simulink model "multidrivesystem"  (R2020a)
settings: Solver=ode23  StartTime=0.0  StopTime=1  MaxStep=20  RelTol=1e-4
libraries: powerlib x250
(part 1 of 2)
settings Model: Creator=shalakasitre  LastModifiedBy=shalakasitre
settings DataIOCC: ReturnWorkspaceOutputs=off

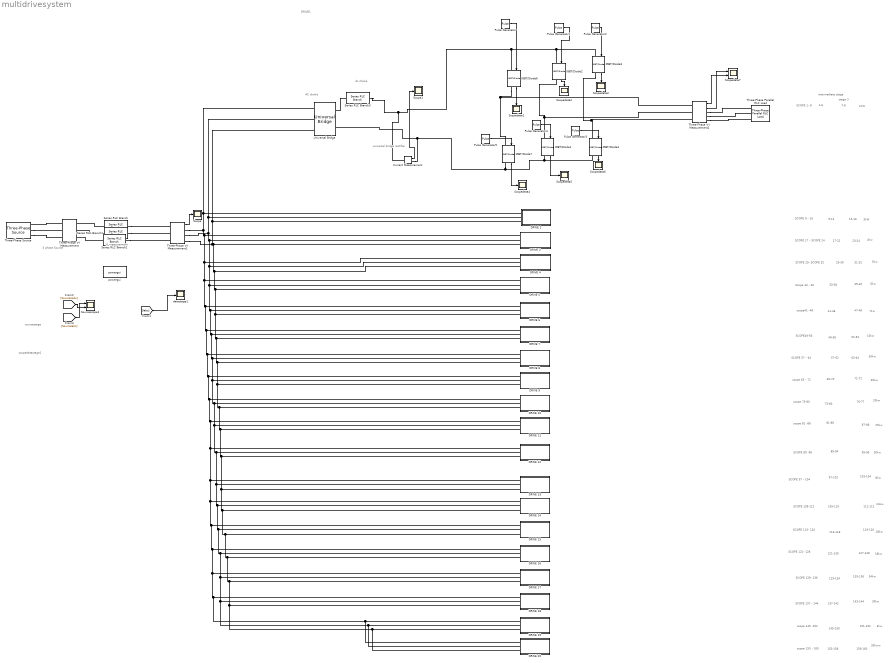
== system multidrivesystem ==
  note: DRIVE1
  note: 30kww
  note: 3kw
  note: 30kw
  note: 34kw
  note: 18kw
  note: 28kw
  note: 24kw
  note: 8kw
  note: 30kw
  note: 25kw
  note: 20kw
  note: 30kw
  note: 30kw
  note: 10kw
  note: 7kw
  note: 6kw
  note: 5kw
  note: 4kw
  note: 3kW
  note: 1kW
  note: 1-6
  note: 153-158
  note: 145-150
  note: 137-142
  note: 129-134
  note: 121-126
  note: 113-118
  note: 105-110
  note: 97-102
  note: 89-94
  note: 81-86
  note: 73-80
  note: 65-70
  note: 57-62
  note: 49-56
  note: 41-46
  note: 33-38
  note: 25-30
  note: 17-22
  note: 9-14
  note: 159-160
  note: 151-152
  note: 143-144
  note: 135-136
  note: 127-128
  note: 119-120
  note: 111-112
  note: 103-104
  note: 95-96
  note: 87-88
  note: 76-77
  note: 71-72
  note: 63-64
  note: 52-53
  note: 47-48
  note: 39-40
  note: 31-32
  note: 23-24
  note: 15-16
  note: intermediate
      | stage
  note: stage 3
  note: sourcestage
  note: scopedatastage1
  note: 7-8
  note: scope 153 - 160
  note: scope 145 -152
  note: SCOPE 137 - 144
  note: SCOPE 129- 136
  note: SCOPE 121- 128
  note: SCOPE 113- 120
  note: SCOPE 105-112
  note: SCOPE 97 - 104
  note: SCOPE 89 -96
  note: scope 81 -88
  note: scope 73-80
  note: scope 65 - 72
  note: SCOPE 57 - 64
  note: scope41- 48
  note: Scope 33 - 40
  note: SCOPE49-56
  note: SCOPE 1- 8
  note: SCOPE 9 - 16
  note: SCOPE 17 - SCOPE 24
  note: SCOPE 25- SCOPE 32
  note: 3 phase Source
  note: VI measurement
  note: universal bridge rectifier
  note: AC choke
  note: dc choke
  Current Measurement : powerlib/Measurements/Current Measurement  PhasorSimulation=off  OutputType=Complex  PSBequivalent=0
  DRIVE 10 : Subsystem
  DRIVE 11 : Subsystem
  DRIVE 12 : Subsystem
  DRIVE 13 : Subsystem
  DRIVE 14 : Subsystem
  DRIVE 15 : Subsystem
  DRIVE 16 : Subsystem
  DRIVE 17 : Subsystem
  DRIVE 18 : Subsystem
  DRIVE 19 : Subsystem
  DRIVE 2 : Subsystem
  DRIVE 20 : Subsystem
  DRIVE 3 : Subsystem
      mask init:
      | set_param(gcb,'LinkStatus','none');
  DRIVE 4 : Subsystem
      mask init:
      | set_param(gcb,'LinkStatus','none');
  DRIVE 5 : Subsystem
  DRIVE 6 : Subsystem
  "DRIVE 7 " : Subsystem
  DRIVE 8 : Subsystem
  DRIVE 9 : Subsystem
  IGBT/Diode{1..4,6..7} (6 alike) : powerlib/Power Electronics/IGBT//Diode  Ron=1e-3  Rs=1e5  Cs=inf  Measurements=on
  Pulse Generator{,1..5} (6 alike) : DiscretePulseGenerator  PulseType=Time based  Period=10  PulseWidth=5
  Scope : Scope
  Scope1 : Scope
  Scopedata{1..6} (6 alike) : Scope
  Scopedata7 : Scope  NumInputPorts=2
  Series RLC Branch : powerlib/Elements/Series RLC Branch  LConnTagsString=__new0  RConnTagsString=__new0  BranchType=L  Resistance=1  Inductance=150e-6  SetiL0=off  InitialCurrent=0  Capacitance=1e-6  Setx0=off  InitialVoltage=0  Measurements=None
  Series RLC Branch1 : powerlib/Elements/Series RLC Branch  LConnTagsString=__new0  RConnTagsString=__new0  BranchType=L  Resistance=1  Inductance=150e-6  SetiL0=off  InitialCurrent=0  Capacitance=1e-6  Setx0=off  InitialVoltage=0  Measurements=None
  Series RLC Branch2 : powerlib/Elements/Series RLC Branch  LConnTagsString=__new0  RConnTagsString=__new0  BranchType=L  Resistance=1  Inductance=150e-6  SetiL0=off  InitialCurrent=0  Capacitance=1e-6  Setx0=off  InitialVoltage=0  Measurements=None
  Series RLC Branch3 : powerlib/Elements/Series RLC Branch  LConnTagsString=__new0  RConnTagsString=__new0  BranchType=L  Resistance=1  Inductance=3e-3  SetiL0=off  InitialCurrent=0  Capacitance=1e-6  Setx0=off  InitialVoltage=0  Measurements=None
  Sourcescope1 : Scope  NumInputPorts=2
  Three-Phase Parallel RLC Load : powerlib/Elements/Three-Phase Parallel RLC Load  LConnTagsString=A|B|C  Configuration=Y (grounded)  NominalVoltage=1000  Vabc=[1e3 1e3 1e3]  Vabcp=[1e3 1e3 1e3]  NominalFrequency=60  UnbalancedPower=off  ActivePower=5e3  InductivePower=0  CapacitivePower=0  Pabc=[10e3 9e3 11e3]  QLabc=[100 90 110]  QCabc=[100 90 110]  Pabcp=[10e3 9e3 11e3]  QLabcp=[100 90 110]  QCabcp=[100 90 110]  Measurements=None  LoadType=constant Z
  Three-Phase V-I Measurement : powerlib/Measurements/Three-Phase V-I Measurement  VoltageMeasurement=phase-to-ground  SetLabelV=on  LabelV=SourceVabc  Vpu=off  VpuLL=off  CurrentMeasurement=yes  SetLabelI=on  LabelI=SourceIabc  Ipu=off  Pbase=100e6  Vbase=500e3  OutputType=Complex  PhasorSimulation=off  PSBequivalent=0
  Three-Phase V-I Measurement1 : powerlib/Measurements/Three-Phase V-I Measurement  VoltageMeasurement=phase-to-ground  SetLabelV=off  LabelV=Vabc  Vpu=off  VpuLL=off  CurrentMeasurement=yes  SetLabelI=on  LabelI=Iabc  Ipu=off  Pbase=100e6  Vbase=500e3  OutputType=Complex  PhasorSimulation=off  PSBequivalent=0
  Three-Phase V-I Measurement2 : powerlib/Measurements/Three-Phase V-I Measurement  VoltageMeasurement=phase-to-ground  SetLabelV=off  LabelV=Vabc  Vpu=off  VpuLL=off  CurrentMeasurement=yes  SetLabelI=off  LabelI=Iabc  Ipu=off  Pbase=100e6  Vbase=500e3  OutputType=Complex  PhasorSimulation=off  PSBequivalent=0
  Three-Phase Source : powerlib/Electrical Sources/Three-Phase Source  InternalConnection=Yg  VoltagePhases=off  Voltage=440  PhaseAngle=0  Voltage_phases=[25e3 25e3 25e3]/sqrt(3)  PhaseAngles_phases=[0 -120 +120]  Frequency=60  NonIdealSource=off  SpecifyImpedance=off  Resistance=0  Inductance=0  ShortCircuitLevel=100e6  BaseVoltage=25e3  XRratio=7  BusType=swing  Pref=10e3  Qref=0  Prefabc=[10e3, 10e3, 10e3]  Qrefabc=[0, 0, 0]  Qmin=-inf  Qmax=inf
  Universal Bridge : powerlib/Power Electronics/Universal Bridge  Arms=3  SnubberResistance=1e5  SnubberCapacitance=inf  Device=Diodes  Ron=1e-3  Lon=0  ForwardVoltages="[  0  0  ]"  ForwardVoltage=0  GTOparameters=[ 10e-6 , 20e-6 ]  IGBTparameters=[ 1e-6 , 2e-6 ]  Measurements=None  Measurements_2=None  converterType=Rectifier
  datastage1 : Scope
  powergui : powerlib/powergui  Priority=1  SimulationMode=Discrete  SampleTime=50e-6  frequency=60  Iterations=50  frequencyindice=0  Pbase=100e6  ErrMax=1e-4  UnitsV=kV  UnitsW=MW  buscounter=0  FunctionMessages=off  echomessages=off  EnableUseOfTLC=off  CurrentSourceSwitches=off  DisableSnubberDevices=off  DisableRonSwitches=off  DisableVfSwitches=off  DisplayEquations=off  AutomaticDiscreteSolvers=off  SolverType=Tustin/Backward Euler (TBE)  Interpol=off  ExternalGateDelay=off  methode=off  Ts=100  x0status=blocks  SPID=on  SwTol=0  HookPort=off  NonlinearTolerance=1e-4  nMaxIteration=100  ContinueOnMaxIteration=off  RestoreLinks=warning  ResistiveCurrentMeasurement=off  Frange=[0:2:500]  Ylog=off  Xlog=on  ShowGrid=off  save=off  variable=ZData  structure=Drive1_stage2voltage  ZoomFFT=off  StartTime=0  cycles=1  DisplayStyle=2  fundamental=60  FreqAxis=off  MaxFrequency=1000  frequencyindicesteady=1  RmsSteady=1  display=off
  wires:
  [Iabc] -> datastage1/1
  [SourceVabc] -> Sourcescope1/2
  [SourceIabc] -> Sourcescope1/1
  Three-Phase V-I Measurement1/1 -> Scope/1
  Three-Phase V-I Measurement2/1 -> Scopedata7/2
  Current Measurement/1 -> Scope1/1
  IGBT/Diode1/1 -> Scopedata5/1
  IGBT/Diode3/1 -> Scopedata3/1
  Pulse Generator1/1 -> IGBT/Diode2/1
  Three-Phase V-I Measurement2/2 -> Scopedata7/1
  Pulse Generator2/1 -> IGBT/Diode3/1
  IGBT/Diode4/1 -> Scopedata6/1
  Pulse Generator5/1 -> IGBT/Diode7/1
  Pulse Generator4/1 -> IGBT/Diode1/1
  IGBT/Diode7/1 -> Scopedata4/1
  IGBT/Diode6/1 -> Scopedata1/1
  IGBT/Diode2/1 -> Scopedata2/1
  Pulse Generator/1 -> IGBT/Diode6/1
  Pulse Generator3/1 -> IGBT/Diode4/1
  connections:
  Three-Phase V-I Measurement/LConn1 -- Three-Phase Source/RConn1
  Three-Phase Source/RConn2 -- Three-Phase V-I Measurement/LConn2
  Three-Phase Source/RConn3 -- Three-Phase V-I Measurement/LConn3
  Series RLC Branch/LConn1 -- Three-Phase V-I Measurement/RConn1
  Series RLC Branch1/LConn1 -- Three-Phase V-I Measurement/RConn2
  Series RLC Branch2/LConn1 -- Three-Phase V-I Measurement/RConn3
  DRIVE 20/LConn3 -- DRIVE 19/LConn3 -- DRIVE 18/LConn3 -- DRIVE 17/LConn3 -- DRIVE 16/LConn3 -- DRIVE 15/LConn3 -- DRIVE 14/LConn3 -- DRIVE 13/LConn3 -- DRIVE 12/LConn3 -- DRIVE 11/LConn3 -- DRIVE 10/LConn3 -- DRIVE 9/LConn3 -- DRIVE 8/LConn3 -- "DRIVE 7 "/LConn3 -- DRIVE 6/LConn3 -- DRIVE 5/LConn3 -- DRIVE 4/LConn3 -- DRIVE 3/LConn3 -- Three-Phase V-I Measurement1/RConn3 -- Universal Bridge/LConn3 -- DRIVE 2/LConn3
  DRIVE 20/LConn1 -- DRIVE 19/LConn1 -- DRIVE 18/LConn1 -- DRIVE 17/LConn1 -- DRIVE 16/LConn1 -- DRIVE 15/LConn1 -- DRIVE 14/LConn1 -- DRIVE 13/LConn1 -- DRIVE 12/LConn1 -- DRIVE 11/LConn1 -- DRIVE 10/LConn1 -- DRIVE 9/LConn1 -- DRIVE 8/LConn1 -- "DRIVE 7 "/LConn1 -- DRIVE 6/LConn1 -- DRIVE 5/LConn1 -- Universal Bridge/LConn1 -- DRIVE 2/LConn1 -- Three-Phase V-I Measurement1/RConn1 -- DRIVE 3/LConn1 -- DRIVE 4/LConn1
  Universal Bridge/LConn2 -- DRIVE 2/LConn2 -- DRIVE 20/LConn2 -- DRIVE 19/LConn2 -- DRIVE 18/LConn2 -- DRIVE 17/LConn2 -- DRIVE 16/LConn2 -- DRIVE 15/LConn2 -- DRIVE 14/LConn2 -- DRIVE 13/LConn2 -- DRIVE 12/LConn2 -- DRIVE 11/LConn2 -- DRIVE 10/LConn2 -- DRIVE 9/LConn2 -- DRIVE 8/LConn2 -- "DRIVE 7 "/LConn2 -- DRIVE 6/LConn2 -- DRIVE 5/LConn2 -- DRIVE 4/LConn2 -- DRIVE 3/LConn2 -- Three-Phase V-I Measurement1/RConn2
  Series RLC Branch/RConn1 -- Three-Phase V-I Measurement1/LConn1
  Series RLC Branch1/RConn1 -- Three-Phase V-I Measurement1/LConn2
  Series RLC Branch2/RConn1 -- Three-Phase V-I Measurement1/LConn3
  Series RLC Branch3/LConn1 -- Universal Bridge/RConn1
  IGBT/Diode3/LConn1 -- Series RLC Branch3/RConn1 -- Current Measurement/LConn1 -- IGBT/Diode6/LConn1 -- IGBT/Diode2/LConn1
  Current Measurement/RConn1 -- IGBT/Diode4/RConn1 -- IGBT/Diode1/RConn1 -- IGBT/Diode7/RConn1 -- Universal Bridge/RConn2
  IGBT/Diode3/RConn1 -- Three-Phase V-I Measurement2/LConn3 -- IGBT/Diode4/LConn1
  Three-Phase V-I Measurement2/RConn1 -- Three-Phase Parallel RLC Load/LConn1
  IGBT/Diode2/RConn1 -- Three-Phase V-I Measurement2/LConn2 -- IGBT/Diode1/LConn1
  IGBT/Diode6/RConn1 -- Three-Phase V-I Measurement2/LConn1 -- IGBT/Diode7/LConn1
  Three-Phase V-I Measurement2/RConn3 -- Three-Phase Parallel RLC Load/LConn3
  Three-Phase V-I Measurement2/RConn2 -- Three-Phase Parallel RLC Load/LConn2

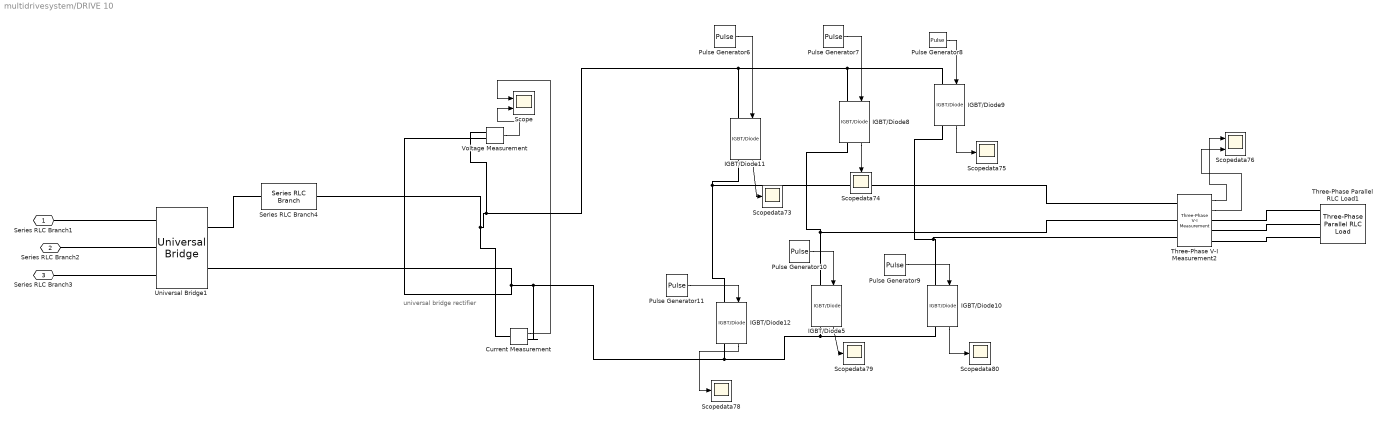
== system multidrivesystem/DRIVE 10 ==
  note: universal bridge rectifier
  Current Measurement : powerlib/Measurements/Current Measurement  PhasorSimulation=off  OutputType=Complex  PSBequivalent=0
  IGBT/Diode{5,8..12} (6 alike) : powerlib/Power Electronics/IGBT//Diode  Ron=1e-3  Rs=1e5  Cs=inf  Measurements=on
  Pulse Generator{6..11} (6 alike) : DiscretePulseGenerator  PulseType=Time based  Period=10  PulseWidth=5
  Scope : Scope  NumInputPorts=2
  Scopedata{73..75,78..80} (6 alike) : Scope
  Scopedata76 : Scope  NumInputPorts=2
  Series RLC Branch4 : powerlib/Elements/Series RLC Branch  LConnTagsString=__new0  RConnTagsString=__new0  BranchType=L  Resistance=1  Inductance=3e-3  SetiL0=off  InitialCurrent=0  Capacitance=1e-6  Setx0=off  InitialVoltage=0  Measurements=None
  Three-Phase Parallel RLC Load1 : powerlib/Elements/Three-Phase Parallel RLC Load  LConnTagsString=A|B|C  Configuration=Y (grounded)  NominalVoltage=1000  Vabc=[1e3 1e3 1e3]  Vabcp=[1e3 1e3 1e3]  NominalFrequency=60  UnbalancedPower=off  ActivePower=9e3  InductivePower=0  CapacitivePower=0  Pabc=[10e3 9e3 11e3]  QLabc=[100 90 110]  QCabc=[100 90 110]  Pabcp=[10e3 9e3 11e3]  QLabcp=[100 90 110]  QCabcp=[100 90 110]  Measurements=None  LoadType=constant Z
  Three-Phase V-I Measurement2 : powerlib/Measurements/Three-Phase V-I Measurement  VoltageMeasurement=phase-to-ground  SetLabelV=off  LabelV=Vabc  Vpu=off  VpuLL=off  CurrentMeasurement=yes  SetLabelI=off  LabelI=Iabc  Ipu=off  Pbase=100e6  Vbase=500e3  OutputType=Complex  PhasorSimulation=off  PSBequivalent=0
  Universal Bridge1 : powerlib/Power Electronics/Universal Bridge  Arms=3  SnubberResistance=1e5  SnubberCapacitance=inf  Device=Diodes  Ron=1e-3  Lon=0  ForwardVoltages="[  0  0  ]"  ForwardVoltage=0  GTOparameters=[ 10e-6 , 20e-6 ]  IGBTparameters=[ 1e-6 , 2e-6 ]  Measurements=None  Measurements_2=None  converterType=Rectifier
  Voltage Measurement : powerlib/Measurements/Voltage Measurement  PhasorSimulation=off  OutputType=Complex  PSBequivalent=0
  Series RLC Branch1 : PMIOPort  Side=Left
  Series RLC Branch2 : PMIOPort  Port=2  Side=Left
  Series RLC Branch3 : PMIOPort  Port=3  Side=Left
  wires:
  IGBT/Diode10/1 -> Scopedata80/1
  IGBT/Diode5/1 -> Scopedata79/1
  IGBT/Diode11/1 -> Scopedata73/1
  IGBT/Diode8/1 -> Scopedata74/1
  IGBT/Diode12/1 -> Scopedata78/1
  Pulse Generator11/1 -> IGBT/Diode12/1
  Pulse Generator8/1 -> IGBT/Diode9/1
  Three-Phase V-I Measurement2/1 -> Scopedata76/1
  Pulse Generator9/1 -> IGBT/Diode10/1
  Pulse Generator7/1 -> IGBT/Diode8/1
  Pulse Generator6/1 -> IGBT/Diode11/1
  Pulse Generator10/1 -> IGBT/Diode5/1
  Three-Phase V-I Measurement2/2 -> Scopedata76/2
  IGBT/Diode9/1 -> Scopedata75/1
  Voltage Measurement/1 -> Scope/2
  Current Measurement/1 -> Scope/1
  connections:
  Three-Phase V-I Measurement2/RConn1 -- Three-Phase Parallel RLC Load1/LConn1
  Three-Phase V-I Measurement2/RConn3 -- Three-Phase Parallel RLC Load1/LConn3
  Three-Phase V-I Measurement2/LConn2 -- IGBT/Diode5/LConn1 -- IGBT/Diode8/RConn1
  Three-Phase V-I Measurement2/RConn2 -- Three-Phase Parallel RLC Load1/LConn2
  IGBT/Diode12/LConn1 -- Three-Phase V-I Measurement2/LConn1 -- IGBT/Diode11/RConn1
  Current Measurement/RConn1 -- IGBT/Diode12/RConn1 -- IGBT/Diode10/RConn1 -- IGBT/Diode5/RConn1 -- Voltage Measurement/LConn2 -- Universal Bridge1/RConn2
  Three-Phase V-I Measurement2/LConn3 -- IGBT/Diode10/LConn1 -- IGBT/Diode9/RConn1
  Voltage Measurement/LConn1 -- Series RLC Branch4/RConn1 -- Current Measurement/LConn1 -- IGBT/Diode9/LConn1 -- IGBT/Diode8/LConn1 -- IGBT/Diode11/LConn1
  Series RLC Branch4/LConn1 -- Universal Bridge1/RConn1
  Universal Bridge1/LConn1 -- Series RLC Branch1/RConn1
  Series RLC Branch2/RConn1 -- Universal Bridge1/LConn2
  Universal Bridge1/LConn3 -- Series RLC Branch3/RConn1

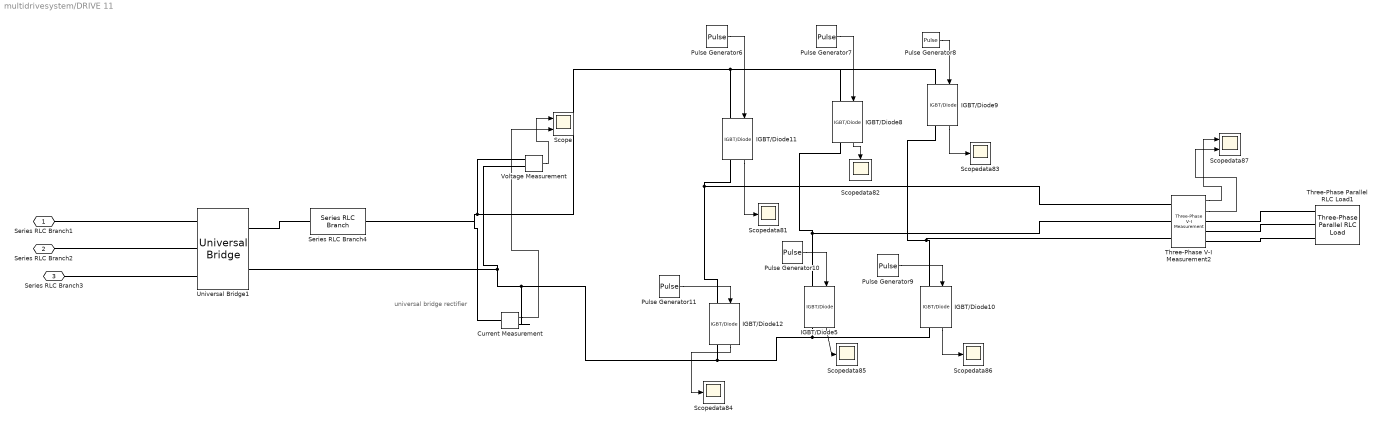
== system multidrivesystem/DRIVE 11 ==
  note: universal bridge rectifier
  Current Measurement : powerlib/Measurements/Current Measurement  PhasorSimulation=off  OutputType=Complex  PSBequivalent=0
  IGBT/Diode{5,8..12} (6 alike) : powerlib/Power Electronics/IGBT//Diode  Ron=1e-3  Rs=1e5  Cs=inf  Measurements=on
  Pulse Generator{6..11} (6 alike) : DiscretePulseGenerator  PulseType=Time based  Period=10  PulseWidth=5
  Scope : Scope  NumInputPorts=2
  Scopedata{81..86} (6 alike) : Scope
  Scopedata87 : Scope  NumInputPorts=2
  Series RLC Branch4 : powerlib/Elements/Series RLC Branch  LConnTagsString=__new0  RConnTagsString=__new0  BranchType=L  Resistance=1  Inductance=3e-3  SetiL0=off  InitialCurrent=0  Capacitance=1e-6  Setx0=off  InitialVoltage=0  Measurements=None
  Three-Phase Parallel RLC Load1 : powerlib/Elements/Three-Phase Parallel RLC Load  LConnTagsString=A|B|C  Configuration=Y (grounded)  NominalVoltage=1000  Vabc=[1e3 1e3 1e3]  Vabcp=[1e3 1e3 1e3]  NominalFrequency=60  UnbalancedPower=off  ActivePower=13e3  InductivePower=0  CapacitivePower=0  Pabc=[10e3 9e3 11e3]  QLabc=[100 90 110]  QCabc=[100 90 110]  Pabcp=[10e3 9e3 11e3]  QLabcp=[100 90 110]  QCabcp=[100 90 110]  Measurements=None  LoadType=constant Z
  Three-Phase V-I Measurement2 : powerlib/Measurements/Three-Phase V-I Measurement  VoltageMeasurement=phase-to-ground  SetLabelV=off  LabelV=Vabc  Vpu=off  VpuLL=off  CurrentMeasurement=yes  SetLabelI=off  LabelI=Iabc  Ipu=off  Pbase=100e6  Vbase=500e3  OutputType=Complex  PhasorSimulation=off  PSBequivalent=0
  Universal Bridge1 : powerlib/Power Electronics/Universal Bridge  Arms=3  SnubberResistance=1e5  SnubberCapacitance=inf  Device=Diodes  Ron=1e-3  Lon=0  ForwardVoltages="[  0  0  ]"  ForwardVoltage=0  GTOparameters=[ 10e-6 , 20e-6 ]  IGBTparameters=[ 1e-6 , 2e-6 ]  Measurements=None  Measurements_2=None  converterType=Rectifier
  Voltage Measurement : powerlib/Measurements/Voltage Measurement  PhasorSimulation=off  OutputType=Complex  PSBequivalent=0
  Series RLC Branch1 : PMIOPort  Side=Left
  Series RLC Branch2 : PMIOPort  Port=2  Side=Left
  Series RLC Branch3 : PMIOPort  Port=3  Side=Left
  wires:
  IGBT/Diode9/1 -> Scopedata83/1
  Three-Phase V-I Measurement2/2 -> Scopedata87/2
  Pulse Generator10/1 -> IGBT/Diode5/1
  Pulse Generator6/1 -> IGBT/Diode11/1
  Pulse Generator7/1 -> IGBT/Diode8/1
  Pulse Generator9/1 -> IGBT/Diode10/1
  Three-Phase V-I Measurement2/1 -> Scopedata87/1
  Pulse Generator8/1 -> IGBT/Diode9/1
  Pulse Generator11/1 -> IGBT/Diode12/1
  IGBT/Diode12/1 -> Scopedata84/1
  IGBT/Diode8/1 -> Scopedata82/1
  IGBT/Diode11/1 -> Scopedata81/1
  IGBT/Diode5/1 -> Scopedata85/1
  IGBT/Diode10/1 -> Scopedata86/1
  Voltage Measurement/1 -> Scope/1
  Current Measurement/1 -> Scope/2
  connections:
  IGBT/Diode9/RConn1 -- IGBT/Diode10/LConn1 -- Three-Phase V-I Measurement2/LConn3
  IGBT/Diode5/RConn1 -- IGBT/Diode10/RConn1 -- IGBT/Diode12/RConn1 -- Current Measurement/RConn1 -- Universal Bridge1/RConn2 -- Voltage Measurement/LConn2
  IGBT/Diode11/RConn1 -- Three-Phase V-I Measurement2/LConn1 -- IGBT/Diode12/LConn1
  Three-Phase V-I Measurement2/RConn2 -- Three-Phase Parallel RLC Load1/LConn2
  IGBT/Diode8/RConn1 -- IGBT/Diode5/LConn1 -- Three-Phase V-I Measurement2/LConn2
  Three-Phase V-I Measurement2/RConn3 -- Three-Phase Parallel RLC Load1/LConn3
  Three-Phase V-I Measurement2/RConn1 -- Three-Phase Parallel RLC Load1/LConn1
  Voltage Measurement/LConn1 -- Series RLC Branch4/RConn1 -- Current Measurement/LConn1 -- IGBT/Diode11/LConn1 -- IGBT/Diode8/LConn1 -- IGBT/Diode9/LConn1
  Series RLC Branch4/LConn1 -- Universal Bridge1/RConn1
  Universal Bridge1/LConn1 -- Series RLC Branch1/RConn1
  Universal Bridge1/LConn2 -- Series RLC Branch2/RConn1
  Series RLC Branch3/RConn1 -- Universal Bridge1/LConn3

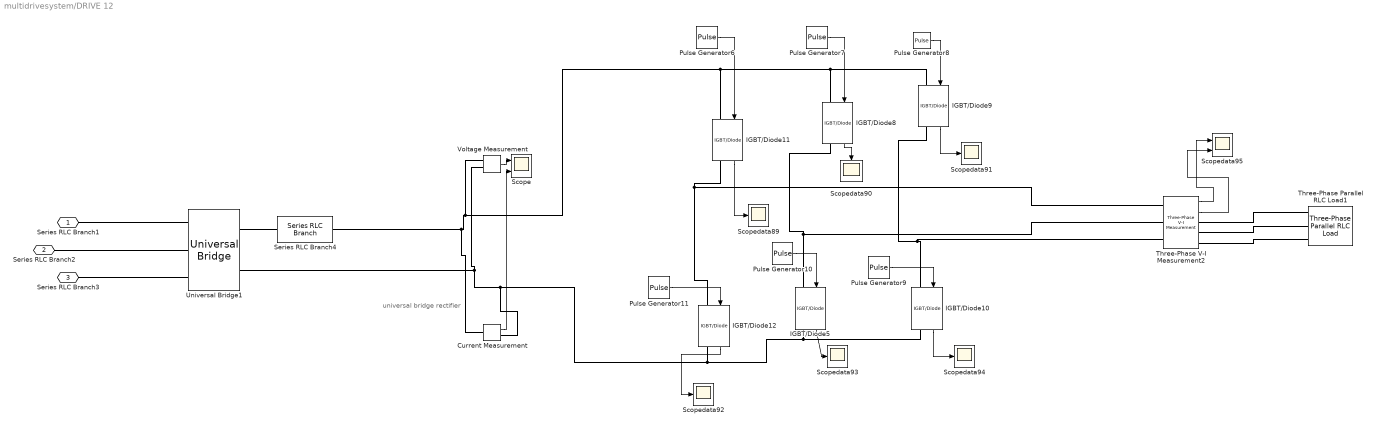
== system multidrivesystem/DRIVE 12 ==
  note: universal bridge rectifier
  Current Measurement : powerlib/Measurements/Current Measurement  PhasorSimulation=off  OutputType=Complex  PSBequivalent=0
  IGBT/Diode{5,8..12} (6 alike) : powerlib/Power Electronics/IGBT//Diode  Ron=1e-3  Rs=1e5  Cs=inf  Measurements=on
  Pulse Generator{6..11} (6 alike) : DiscretePulseGenerator  PulseType=Time based  Period=10  PulseWidth=5
  Scope : Scope  NumInputPorts=2
  Scopedata{89..94} (6 alike) : Scope
  Scopedata95 : Scope  NumInputPorts=2
  Series RLC Branch4 : powerlib/Elements/Series RLC Branch  LConnTagsString=__new0  RConnTagsString=__new0  BranchType=L  Resistance=1  Inductance=3e-3  SetiL0=off  InitialCurrent=0  Capacitance=1e-6  Setx0=off  InitialVoltage=0  Measurements=None
  Three-Phase Parallel RLC Load1 : powerlib/Elements/Three-Phase Parallel RLC Load  LConnTagsString=A|B|C  Configuration=Y (grounded)  NominalVoltage=1000  Vabc=[1e3 1e3 1e3]  Vabcp=[1e3 1e3 1e3]  NominalFrequency=60  UnbalancedPower=off  ActivePower=1e3  InductivePower=0  CapacitivePower=0  Pabc=[10e3 9e3 11e3]  QLabc=[100 90 110]  QCabc=[100 90 110]  Pabcp=[10e3 9e3 11e3]  QLabcp=[100 90 110]  QCabcp=[100 90 110]  Measurements=None  LoadType=constant Z
  Three-Phase V-I Measurement2 : powerlib/Measurements/Three-Phase V-I Measurement  VoltageMeasurement=phase-to-ground  SetLabelV=off  LabelV=Vabc  Vpu=off  VpuLL=off  CurrentMeasurement=yes  SetLabelI=off  LabelI=Iabc  Ipu=off  Pbase=100e6  Vbase=500e3  OutputType=Complex  PhasorSimulation=off  PSBequivalent=0
  Universal Bridge1 : powerlib/Power Electronics/Universal Bridge  Arms=3  SnubberResistance=1e5  SnubberCapacitance=inf  Device=Diodes  Ron=1e-3  Lon=0  ForwardVoltages="[  0  0  ]"  ForwardVoltage=0  GTOparameters=[ 10e-6 , 20e-6 ]  IGBTparameters=[ 1e-6 , 2e-6 ]  Measurements=None  Measurements_2=None  converterType=Rectifier
  Voltage Measurement : powerlib/Measurements/Voltage Measurement  PhasorSimulation=off  OutputType=Complex  PSBequivalent=0
  Series RLC Branch1 : PMIOPort  Side=Left
  Series RLC Branch2 : PMIOPort  Port=2  Side=Left
  Series RLC Branch3 : PMIOPort  Port=3  Side=Left
  wires:
  IGBT/Diode10/1 -> Scopedata94/1
  IGBT/Diode5/1 -> Scopedata93/1
  IGBT/Diode11/1 -> Scopedata89/1
  IGBT/Diode8/1 -> Scopedata90/1
  IGBT/Diode12/1 -> Scopedata92/1
  Pulse Generator11/1 -> IGBT/Diode12/1
  Pulse Generator8/1 -> IGBT/Diode9/1
  Three-Phase V-I Measurement2/1 -> Scopedata95/1
  Pulse Generator9/1 -> IGBT/Diode10/1
  Pulse Generator7/1 -> IGBT/Diode8/1
  Pulse Generator6/1 -> IGBT/Diode11/1
  Pulse Generator10/1 -> IGBT/Diode5/1
  Three-Phase V-I Measurement2/2 -> Scopedata95/2
  IGBT/Diode9/1 -> Scopedata91/1
  Voltage Measurement/1 -> Scope/1
  Current Measurement/1 -> Scope/2
  connections:
  Three-Phase V-I Measurement2/RConn1 -- Three-Phase Parallel RLC Load1/LConn1
  Three-Phase V-I Measurement2/RConn3 -- Three-Phase Parallel RLC Load1/LConn3
  Three-Phase V-I Measurement2/LConn2 -- IGBT/Diode5/LConn1 -- IGBT/Diode8/RConn1
  Three-Phase V-I Measurement2/RConn2 -- Three-Phase Parallel RLC Load1/LConn2
  IGBT/Diode12/LConn1 -- Three-Phase V-I Measurement2/LConn1 -- IGBT/Diode11/RConn1
  Current Measurement/RConn1 -- IGBT/Diode12/RConn1 -- IGBT/Diode10/RConn1 -- IGBT/Diode5/RConn1 -- Voltage Measurement/LConn2 -- Universal Bridge1/RConn2
  Three-Phase V-I Measurement2/LConn3 -- IGBT/Diode10/LConn1 -- IGBT/Diode9/RConn1
  Voltage Measurement/LConn1 -- Series RLC Branch4/RConn1 -- Current Measurement/LConn1 -- IGBT/Diode9/LConn1 -- IGBT/Diode8/LConn1 -- IGBT/Diode11/LConn1
  Series RLC Branch4/LConn1 -- Universal Bridge1/RConn1
  Series RLC Branch1/RConn1 -- Universal Bridge1/LConn1
  Universal Bridge1/LConn2 -- Series RLC Branch2/RConn1
  Universal Bridge1/LConn3 -- Series RLC Branch3/RConn1

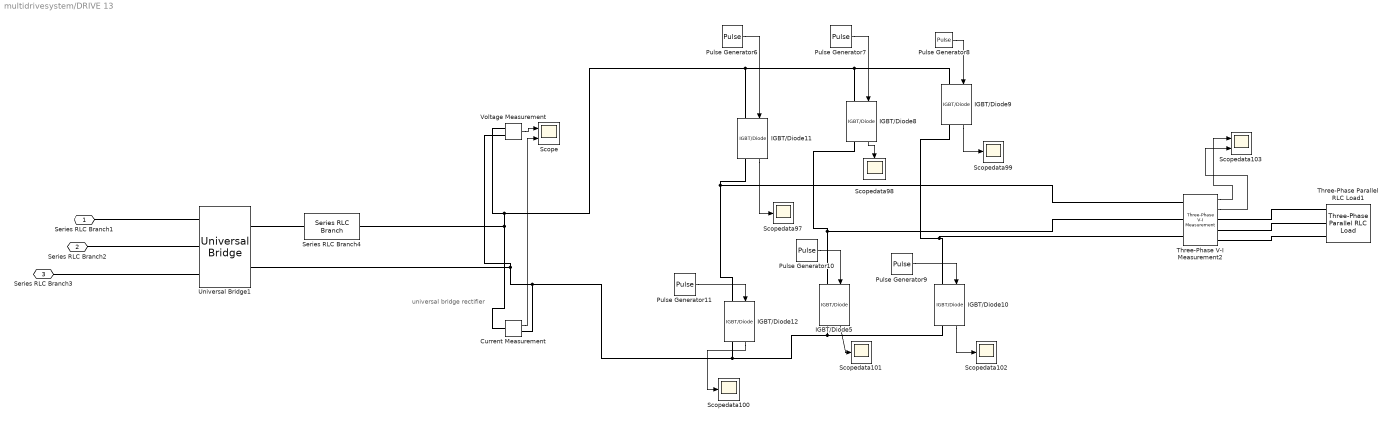
== system multidrivesystem/DRIVE 13 ==
  note: universal bridge rectifier
  Current Measurement : powerlib/Measurements/Current Measurement  PhasorSimulation=off  OutputType=Complex  PSBequivalent=0
  IGBT/Diode{5,8..12} (6 alike) : powerlib/Power Electronics/IGBT//Diode  Ron=1e-3  Rs=1e5  Cs=inf  Measurements=on
  Pulse Generator{6..11} (6 alike) : DiscretePulseGenerator  PulseType=Time based  Period=10  PulseWidth=5
  Scope : Scope  NumInputPorts=2
  Scopedata{97..102} (6 alike) : Scope
  Scopedata103 : Scope  NumInputPorts=2
  Series RLC Branch4 : powerlib/Elements/Series RLC Branch  LConnTagsString=__new0  RConnTagsString=__new0  BranchType=L  Resistance=1  Inductance=3e-3  SetiL0=off  InitialCurrent=0  Capacitance=1e-6  Setx0=off  InitialVoltage=0  Measurements=None
  Three-Phase Parallel RLC Load1 : powerlib/Elements/Three-Phase Parallel RLC Load  LConnTagsString=A|B|C  Configuration=Y (grounded)  NominalVoltage=1000  Vabc=[1e3 1e3 1e3]  Vabcp=[1e3 1e3 1e3]  NominalFrequency=60  UnbalancedPower=off  ActivePower=6e3  InductivePower=0  CapacitivePower=0  Pabc=[10e3 9e3 11e3]  QLabc=[100 90 110]  QCabc=[100 90 110]  Pabcp=[10e3 9e3 11e3]  QLabcp=[100 90 110]  QCabcp=[100 90 110]  Measurements=None  LoadType=constant Z
  Three-Phase V-I Measurement2 : powerlib/Measurements/Three-Phase V-I Measurement  VoltageMeasurement=phase-to-ground  SetLabelV=off  LabelV=Vabc  Vpu=off  VpuLL=off  CurrentMeasurement=yes  SetLabelI=off  LabelI=Iabc  Ipu=off  Pbase=100e6  Vbase=500e3  OutputType=Complex  PhasorSimulation=off  PSBequivalent=0
  Universal Bridge1 : powerlib/Power Electronics/Universal Bridge  Arms=3  SnubberResistance=1e5  SnubberCapacitance=inf  Device=Diodes  Ron=1e-3  Lon=0  ForwardVoltages="[  0  0  ]"  ForwardVoltage=0  GTOparameters=[ 10e-6 , 20e-6 ]  IGBTparameters=[ 1e-6 , 2e-6 ]  Measurements=None  Measurements_2=None  converterType=Rectifier
  Voltage Measurement : powerlib/Measurements/Voltage Measurement  PhasorSimulation=off  OutputType=Complex  PSBequivalent=0
  Series RLC Branch1 : PMIOPort  Side=Left
  Series RLC Branch2 : PMIOPort  Port=2  Side=Left
  Series RLC Branch3 : PMIOPort  Port=3  Side=Left
  wires:
  IGBT/Diode9/1 -> Scopedata99/1
  Three-Phase V-I Measurement2/2 -> Scopedata103/2
  Pulse Generator10/1 -> IGBT/Diode5/1
  Pulse Generator6/1 -> IGBT/Diode11/1
  Pulse Generator7/1 -> IGBT/Diode8/1
  Pulse Generator9/1 -> IGBT/Diode10/1
  Three-Phase V-I Measurement2/1 -> Scopedata103/1
  Pulse Generator8/1 -> IGBT/Diode9/1
  Pulse Generator11/1 -> IGBT/Diode12/1
  IGBT/Diode12/1 -> Scopedata100/1
  IGBT/Diode8/1 -> Scopedata98/1
  IGBT/Diode11/1 -> Scopedata97/1
  IGBT/Diode5/1 -> Scopedata101/1
  IGBT/Diode10/1 -> Scopedata102/1
  Voltage Measurement/1 -> Scope/1
  Current Measurement/1 -> Scope/2
  connections:
  IGBT/Diode9/RConn1 -- IGBT/Diode10/LConn1 -- Three-Phase V-I Measurement2/LConn3
  IGBT/Diode5/RConn1 -- IGBT/Diode10/RConn1 -- IGBT/Diode12/RConn1 -- Current Measurement/RConn1 -- Voltage Measurement/LConn2 -- Universal Bridge1/RConn2
  IGBT/Diode11/RConn1 -- Three-Phase V-I Measurement2/LConn1 -- IGBT/Diode12/LConn1
  Three-Phase V-I Measurement2/RConn2 -- Three-Phase Parallel RLC Load1/LConn2
  IGBT/Diode8/RConn1 -- IGBT/Diode5/LConn1 -- Three-Phase V-I Measurement2/LConn2
  Three-Phase V-I Measurement2/RConn3 -- Three-Phase Parallel RLC Load1/LConn3
  Three-Phase V-I Measurement2/RConn1 -- Three-Phase Parallel RLC Load1/LConn1
  Series RLC Branch4/RConn1 -- Current Measurement/LConn1 -- Voltage Measurement/LConn1 -- IGBT/Diode11/LConn1 -- IGBT/Diode8/LConn1 -- IGBT/Diode9/LConn1
  Series RLC Branch4/LConn1 -- Universal Bridge1/RConn1
  Universal Bridge1/LConn1 -- Series RLC Branch1/RConn1
  Universal Bridge1/LConn2 -- Series RLC Branch2/RConn1
  Universal Bridge1/LConn3 -- Series RLC Branch3/RConn1

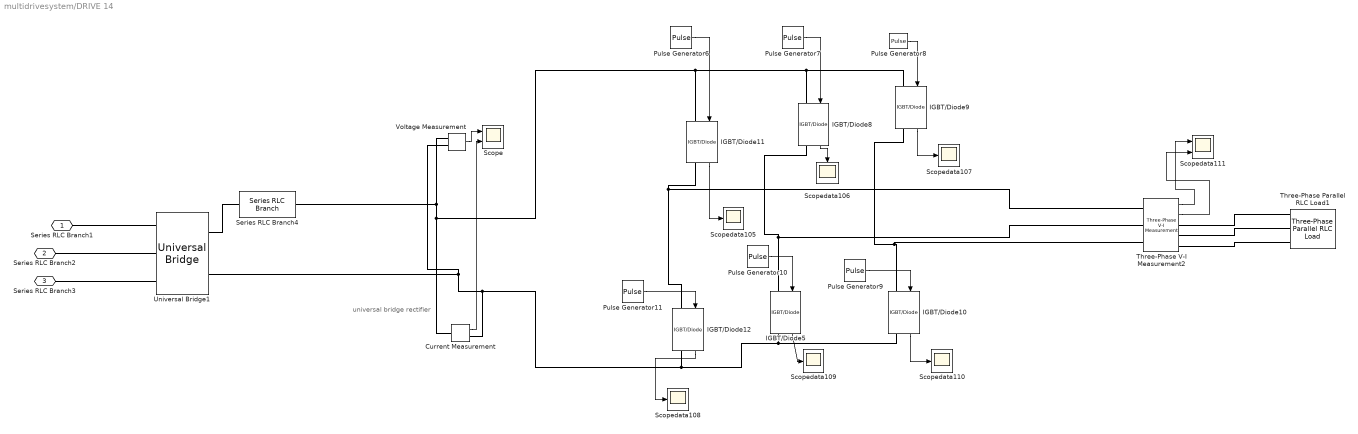
== system multidrivesystem/DRIVE 14 ==
  note: universal bridge rectifier
  Current Measurement : powerlib/Measurements/Current Measurement  PhasorSimulation=off  OutputType=Complex  PSBequivalent=0
  IGBT/Diode{5,8..12} (6 alike) : powerlib/Power Electronics/IGBT//Diode  Ron=1e-3  Rs=1e5  Cs=inf  Measurements=on
  Pulse Generator{6..11} (6 alike) : DiscretePulseGenerator  PulseType=Time based  Period=10  PulseWidth=5
  Scope : Scope  NumInputPorts=2
  Scopedata{105..110} (6 alike) : Scope
  Scopedata111 : Scope  NumInputPorts=2
  Series RLC Branch4 : powerlib/Elements/Series RLC Branch  LConnTagsString=__new0  RConnTagsString=__new0  BranchType=L  Resistance=1  Inductance=3e-3  SetiL0=off  InitialCurrent=0  Capacitance=1e-6  Setx0=off  InitialVoltage=0  Measurements=None
  Three-Phase Parallel RLC Load1 : powerlib/Elements/Three-Phase Parallel RLC Load  LConnTagsString=A|B|C  Configuration=Y (grounded)  NominalVoltage=1000  Vabc=[1e3 1e3 1e3]  Vabcp=[1e3 1e3 1e3]  NominalFrequency=60  UnbalancedPower=off  ActivePower=7e3  InductivePower=0  CapacitivePower=0  Pabc=[10e3 9e3 11e3]  QLabc=[100 90 110]  QCabc=[100 90 110]  Pabcp=[10e3 9e3 11e3]  QLabcp=[100 90 110]  QCabcp=[100 90 110]  Measurements=None  LoadType=constant Z
  Three-Phase V-I Measurement2 : powerlib/Measurements/Three-Phase V-I Measurement  VoltageMeasurement=phase-to-ground  SetLabelV=off  LabelV=Vabc  Vpu=off  VpuLL=off  CurrentMeasurement=yes  SetLabelI=off  LabelI=Iabc  Ipu=off  Pbase=100e6  Vbase=500e3  OutputType=Complex  PhasorSimulation=off  PSBequivalent=0
  Universal Bridge1 : powerlib/Power Electronics/Universal Bridge  Arms=3  SnubberResistance=1e5  SnubberCapacitance=inf  Device=Diodes  Ron=1e-3  Lon=0  ForwardVoltages="[  0  0  ]"  ForwardVoltage=0  GTOparameters=[ 10e-6 , 20e-6 ]  IGBTparameters=[ 1e-6 , 2e-6 ]  Measurements=None  Measurements_2=None  converterType=Rectifier
  Voltage Measurement : powerlib/Measurements/Voltage Measurement  PhasorSimulation=off  OutputType=Complex  PSBequivalent=0
  Series RLC Branch1 : PMIOPort  Side=Left
  Series RLC Branch2 : PMIOPort  Port=2  Side=Left
  Series RLC Branch3 : PMIOPort  Port=3  Side=Left
  wires:
  IGBT/Diode10/1 -> Scopedata110/1
  IGBT/Diode5/1 -> Scopedata109/1
  IGBT/Diode11/1 -> Scopedata105/1
  IGBT/Diode8/1 -> Scopedata106/1
  IGBT/Diode12/1 -> Scopedata108/1
  Pulse Generator11/1 -> IGBT/Diode12/1
  Pulse Generator8/1 -> IGBT/Diode9/1
  Three-Phase V-I Measurement2/1 -> Scopedata111/1
  Pulse Generator9/1 -> IGBT/Diode10/1
  Pulse Generator7/1 -> IGBT/Diode8/1
  Pulse Generator6/1 -> IGBT/Diode11/1
  Pulse Generator10/1 -> IGBT/Diode5/1
  Three-Phase V-I Measurement2/2 -> Scopedata111/2
  IGBT/Diode9/1 -> Scopedata107/1
  Voltage Measurement/1 -> Scope/1
  Current Measurement/1 -> Scope/2
  connections:
  Three-Phase V-I Measurement2/RConn1 -- Three-Phase Parallel RLC Load1/LConn1
  Three-Phase V-I Measurement2/RConn3 -- Three-Phase Parallel RLC Load1/LConn3
  Three-Phase V-I Measurement2/LConn2 -- IGBT/Diode5/LConn1 -- IGBT/Diode8/RConn1
  Three-Phase V-I Measurement2/RConn2 -- Three-Phase Parallel RLC Load1/LConn2
  IGBT/Diode12/LConn1 -- Three-Phase V-I Measurement2/LConn1 -- IGBT/Diode11/RConn1
  Current Measurement/RConn1 -- IGBT/Diode12/RConn1 -- IGBT/Diode10/RConn1 -- IGBT/Diode5/RConn1 -- Voltage Measurement/LConn2 -- Universal Bridge1/RConn2
  Three-Phase V-I Measurement2/LConn3 -- IGBT/Diode10/LConn1 -- IGBT/Diode9/RConn1
  Voltage Measurement/LConn1 -- Series RLC Branch4/RConn1 -- Current Measurement/LConn1 -- IGBT/Diode9/LConn1 -- IGBT/Diode8/LConn1 -- IGBT/Diode11/LConn1
  Series RLC Branch4/LConn1 -- Universal Bridge1/RConn1
  Universal Bridge1/LConn1 -- Series RLC Branch1/RConn1
  Series RLC Branch2/RConn1 -- Universal Bridge1/LConn2
  Series RLC Branch3/RConn1 -- Universal Bridge1/LConn3

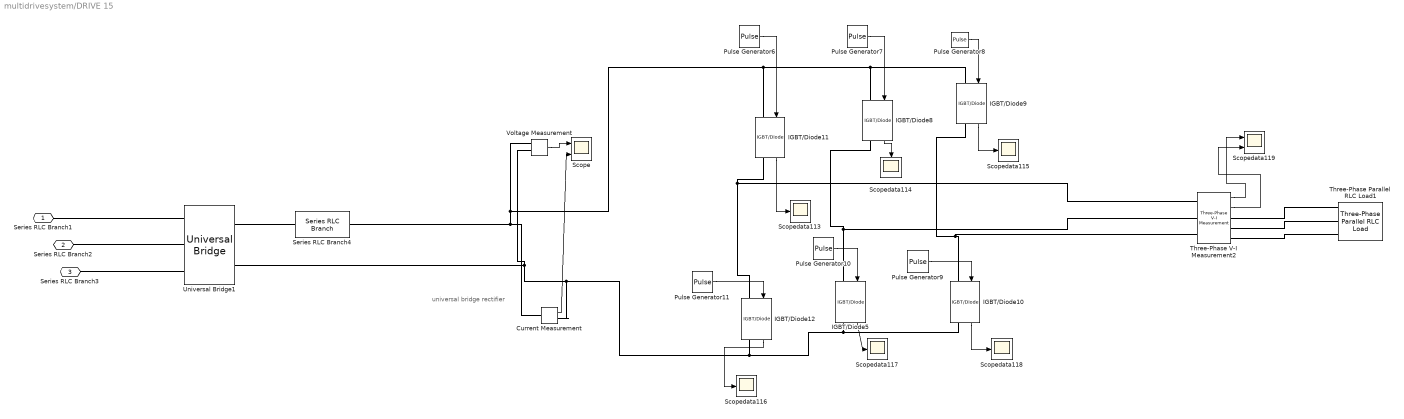
== system multidrivesystem/DRIVE 15 ==
  note: universal bridge rectifier
  Current Measurement : powerlib/Measurements/Current Measurement  PhasorSimulation=off  OutputType=Complex  PSBequivalent=0
  IGBT/Diode{5,8..12} (6 alike) : powerlib/Power Electronics/IGBT//Diode  Ron=1e-3  Rs=1e5  Cs=inf  Measurements=on
  Pulse Generator{6..11} (6 alike) : DiscretePulseGenerator  PulseType=Time based  Period=10  PulseWidth=5
  Scope : Scope  NumInputPorts=2
  Scopedata{113..118} (6 alike) : Scope
  Scopedata119 : Scope  NumInputPorts=2
  Series RLC Branch4 : powerlib/Elements/Series RLC Branch  LConnTagsString=__new0  RConnTagsString=__new0  BranchType=L  Resistance=1  Inductance=3e-3  SetiL0=off  InitialCurrent=0  Capacitance=1e-6  Setx0=off  InitialVoltage=0  Measurements=None
  Three-Phase Parallel RLC Load1 : powerlib/Elements/Three-Phase Parallel RLC Load  LConnTagsString=A|B|C  Configuration=Y (grounded)  NominalVoltage=1000  Vabc=[1e3 1e3 1e3]  Vabcp=[1e3 1e3 1e3]  NominalFrequency=60  UnbalancedPower=off  ActivePower=5e3  InductivePower=0  CapacitivePower=0  Pabc=[10e3 9e3 11e3]  QLabc=[100 90 110]  QCabc=[100 90 110]  Pabcp=[10e3 9e3 11e3]  QLabcp=[100 90 110]  QCabcp=[100 90 110]  Measurements=None  LoadType=constant Z
  Three-Phase V-I Measurement2 : powerlib/Measurements/Three-Phase V-I Measurement  VoltageMeasurement=phase-to-ground  SetLabelV=off  LabelV=Vabc  Vpu=off  VpuLL=off  CurrentMeasurement=yes  SetLabelI=off  LabelI=Iabc  Ipu=off  Pbase=100e6  Vbase=500e3  OutputType=Complex  PhasorSimulation=off  PSBequivalent=0
  Universal Bridge1 : powerlib/Power Electronics/Universal Bridge  Arms=3  SnubberResistance=1e5  SnubberCapacitance=inf  Device=Diodes  Ron=1e-3  Lon=0  ForwardVoltages="[  0  0  ]"  ForwardVoltage=0  GTOparameters=[ 10e-6 , 20e-6 ]  IGBTparameters=[ 1e-6 , 2e-6 ]  Measurements=None  Measurements_2=None  converterType=Rectifier
  Voltage Measurement : powerlib/Measurements/Voltage Measurement  PhasorSimulation=off  OutputType=Complex  PSBequivalent=0
  Series RLC Branch1 : PMIOPort  Side=Left
  Series RLC Branch2 : PMIOPort  Port=2  Side=Left
  Series RLC Branch3 : PMIOPort  Port=3  Side=Left
  wires:
  IGBT/Diode9/1 -> Scopedata115/1
  Three-Phase V-I Measurement2/2 -> Scopedata119/2
  Pulse Generator10/1 -> IGBT/Diode5/1
  Pulse Generator6/1 -> IGBT/Diode11/1
  Pulse Generator7/1 -> IGBT/Diode8/1
  Pulse Generator9/1 -> IGBT/Diode10/1
  Three-Phase V-I Measurement2/1 -> Scopedata119/1
  Pulse Generator8/1 -> IGBT/Diode9/1
  Pulse Generator11/1 -> IGBT/Diode12/1
  IGBT/Diode12/1 -> Scopedata116/1
  IGBT/Diode8/1 -> Scopedata114/1
  IGBT/Diode11/1 -> Scopedata113/1
  IGBT/Diode5/1 -> Scopedata117/1
  IGBT/Diode10/1 -> Scopedata118/1
  Voltage Measurement/1 -> Scope/1
  Current Measurement/1 -> Scope/2
  connections:
  IGBT/Diode9/RConn1 -- IGBT/Diode10/LConn1 -- Three-Phase V-I Measurement2/LConn3
  IGBT/Diode5/RConn1 -- IGBT/Diode10/RConn1 -- IGBT/Diode12/RConn1 -- Current Measurement/RConn1 -- Universal Bridge1/RConn2 -- Voltage Measurement/LConn2
  IGBT/Diode11/RConn1 -- Three-Phase V-I Measurement2/LConn1 -- IGBT/Diode12/LConn1
  Three-Phase V-I Measurement2/RConn2 -- Three-Phase Parallel RLC Load1/LConn2
  IGBT/Diode8/RConn1 -- IGBT/Diode5/LConn1 -- Three-Phase V-I Measurement2/LConn2
  Three-Phase V-I Measurement2/RConn3 -- Three-Phase Parallel RLC Load1/LConn3
  Three-Phase V-I Measurement2/RConn1 -- Three-Phase Parallel RLC Load1/LConn1
  Series RLC Branch4/RConn1 -- Current Measurement/LConn1 -- Voltage Measurement/LConn1 -- IGBT/Diode11/LConn1 -- IGBT/Diode8/LConn1 -- IGBT/Diode9/LConn1
  Series RLC Branch4/LConn1 -- Universal Bridge1/RConn1
  Series RLC Branch1/RConn1 -- Universal Bridge1/LConn1
  Series RLC Branch2/RConn1 -- Universal Bridge1/LConn2
  Universal Bridge1/LConn3 -- Series RLC Branch3/RConn1

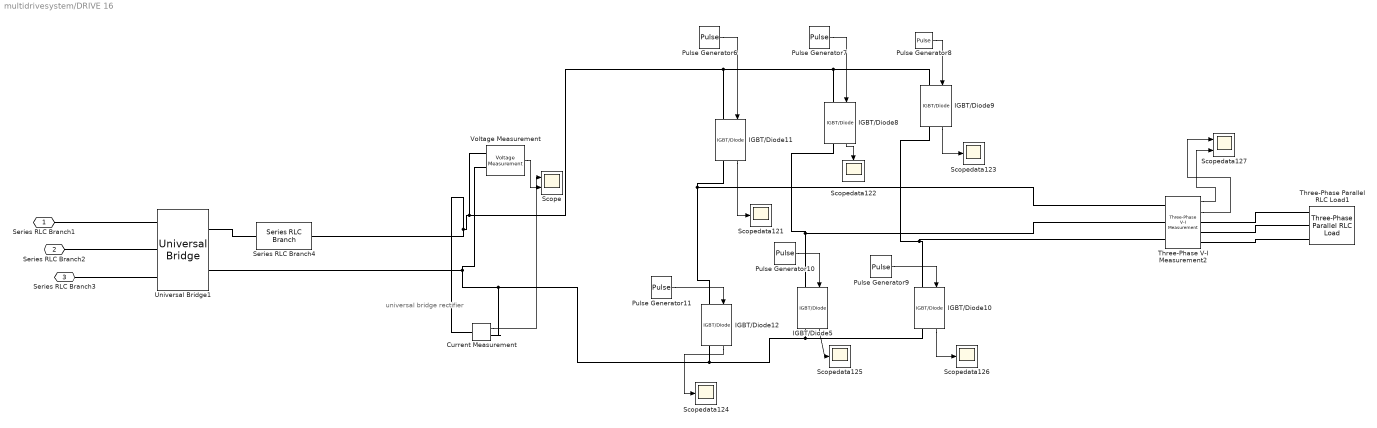
== system multidrivesystem/DRIVE 16 ==
  note: universal bridge rectifier
  Current Measurement : powerlib/Measurements/Current Measurement  PhasorSimulation=off  OutputType=Complex  PSBequivalent=0
  IGBT/Diode{5,8..12} (6 alike) : powerlib/Power Electronics/IGBT//Diode  Ron=1e-3  Rs=1e5  Cs=inf  Measurements=on
  Pulse Generator{6..11} (6 alike) : DiscretePulseGenerator  PulseType=Time based  Period=10  PulseWidth=5
  Scope : Scope  NumInputPorts=2
  Scopedata{121..126} (6 alike) : Scope
  Scopedata127 : Scope  NumInputPorts=2
  Series RLC Branch4 : powerlib/Elements/Series RLC Branch  LConnTagsString=__new0  RConnTagsString=__new0  BranchType=L  Resistance=1  Inductance=3e-3  SetiL0=off  InitialCurrent=0  Capacitance=1e-6  Setx0=off  InitialVoltage=0  Measurements=None
  Three-Phase Parallel RLC Load1 : powerlib/Elements/Three-Phase Parallel RLC Load  LConnTagsString=A|B|C  Configuration=Y (grounded)  NominalVoltage=1000  Vabc=[1e3 1e3 1e3]  Vabcp=[1e3 1e3 1e3]  NominalFrequency=60  UnbalancedPower=off  ActivePower=3e3  InductivePower=0  CapacitivePower=0  Pabc=[10e3 9e3 11e3]  QLabc=[100 90 110]  QCabc=[100 90 110]  Pabcp=[10e3 9e3 11e3]  QLabcp=[100 90 110]  QCabcp=[100 90 110]  Measurements=None  LoadType=constant Z
  Three-Phase V-I Measurement2 : powerlib/Measurements/Three-Phase V-I Measurement  VoltageMeasurement=phase-to-ground  SetLabelV=off  LabelV=Vabc  Vpu=off  VpuLL=off  CurrentMeasurement=yes  SetLabelI=off  LabelI=Iabc  Ipu=off  Pbase=100e6  Vbase=500e3  OutputType=Complex  PhasorSimulation=off  PSBequivalent=0
  Universal Bridge1 : powerlib/Power Electronics/Universal Bridge  Arms=3  SnubberResistance=1e5  SnubberCapacitance=inf  Device=Diodes  Ron=1e-3  Lon=0  ForwardVoltages="[  0  0  ]"  ForwardVoltage=0  GTOparameters=[ 10e-6 , 20e-6 ]  IGBTparameters=[ 1e-6 , 2e-6 ]  Measurements=None  Measurements_2=None  converterType=Rectifier
  Voltage Measurement : powerlib/Measurements/Voltage Measurement  PhasorSimulation=off  OutputType=Complex  PSBequivalent=0
  Series RLC Branch1 : PMIOPort  Side=Left
  Series RLC Branch2 : PMIOPort  Port=2  Side=Left
  Series RLC Branch3 : PMIOPort  Port=3  Side=Left
  wires:
  IGBT/Diode10/1 -> Scopedata126/1
  IGBT/Diode5/1 -> Scopedata125/1
  IGBT/Diode11/1 -> Scopedata121/1
  IGBT/Diode8/1 -> Scopedata122/1
  IGBT/Diode12/1 -> Scopedata124/1
  Pulse Generator11/1 -> IGBT/Diode12/1
  Pulse Generator8/1 -> IGBT/Diode9/1
  Three-Phase V-I Measurement2/1 -> Scopedata127/2
  Pulse Generator9/1 -> IGBT/Diode10/1
  Pulse Generator7/1 -> IGBT/Diode8/1
  Pulse Generator6/1 -> IGBT/Diode11/1
  Pulse Generator10/1 -> IGBT/Diode5/1
  Three-Phase V-I Measurement2/2 -> Scopedata127/1
  IGBT/Diode9/1 -> Scopedata123/1
  Voltage Measurement/1 -> Scope/2
  Current Measurement/1 -> Scope/1
  connections:
  Three-Phase V-I Measurement2/RConn1 -- Three-Phase Parallel RLC Load1/LConn1
  Three-Phase V-I Measurement2/RConn3 -- Three-Phase Parallel RLC Load1/LConn3
  Three-Phase V-I Measurement2/LConn2 -- IGBT/Diode5/LConn1 -- IGBT/Diode8/RConn1
  Three-Phase V-I Measurement2/RConn2 -- Three-Phase Parallel RLC Load1/LConn2
  IGBT/Diode12/LConn1 -- Three-Phase V-I Measurement2/LConn1 -- IGBT/Diode11/RConn1
  Current Measurement/RConn1 -- IGBT/Diode12/RConn1 -- IGBT/Diode10/RConn1 -- IGBT/Diode5/RConn1 -- Universal Bridge1/RConn2 -- Voltage Measurement/LConn2
  Three-Phase V-I Measurement2/LConn3 -- IGBT/Diode10/LConn1 -- IGBT/Diode9/RConn1
  Voltage Measurement/LConn1 -- Series RLC Branch4/RConn1 -- Current Measurement/LConn1 -- IGBT/Diode9/LConn1 -- IGBT/Diode8/LConn1 -- IGBT/Diode11/LConn1
  Series RLC Branch4/LConn1 -- Universal Bridge1/RConn1
  Universal Bridge1/LConn1 -- Series RLC Branch1/RConn1
  Universal Bridge1/LConn2 -- Series RLC Branch2/RConn1
  Series RLC Branch3/RConn1 -- Universal Bridge1/LConn3

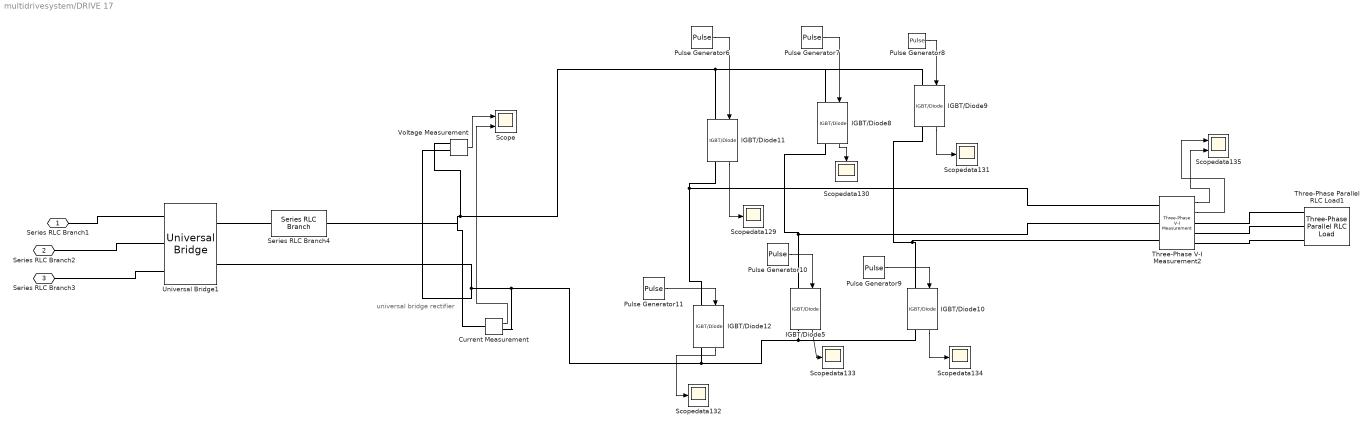
== system multidrivesystem/DRIVE 17 ==
  note: universal bridge rectifier
  Current Measurement : powerlib/Measurements/Current Measurement  PhasorSimulation=off  OutputType=Complex  PSBequivalent=0
  IGBT/Diode{5,8..12} (6 alike) : powerlib/Power Electronics/IGBT//Diode  Ron=1e-3  Rs=1e5  Cs=inf  Measurements=on
  Pulse Generator{6..11} (6 alike) : DiscretePulseGenerator  PulseType=Time based  Period=10  PulseWidth=5
  Scope : Scope  NumInputPorts=2
  Scopedata{129..134} (6 alike) : Scope
  Scopedata135 : Scope  NumInputPorts=2
  Series RLC Branch4 : powerlib/Elements/Series RLC Branch  LConnTagsString=__new0  RConnTagsString=__new0  BranchType=L  Resistance=1  Inductance=3e-3  SetiL0=off  InitialCurrent=0  Capacitance=1e-6  Setx0=off  InitialVoltage=0  Measurements=None
  Three-Phase Parallel RLC Load1 : powerlib/Elements/Three-Phase Parallel RLC Load  LConnTagsString=A|B|C  Configuration=Y (grounded)  NominalVoltage=1000  Vabc=[1e3 1e3 1e3]  Vabcp=[1e3 1e3 1e3]  NominalFrequency=60  UnbalancedPower=off  ActivePower=5e3  InductivePower=0  CapacitivePower=0  Pabc=[10e3 9e3 11e3]  QLabc=[100 90 110]  QCabc=[100 90 110]  Pabcp=[10e3 9e3 11e3]  QLabcp=[100 90 110]  QCabcp=[100 90 110]  Measurements=None  LoadType=constant Z
  Three-Phase V-I Measurement2 : powerlib/Measurements/Three-Phase V-I Measurement  VoltageMeasurement=phase-to-ground  SetLabelV=off  LabelV=Vabc  Vpu=off  VpuLL=off  CurrentMeasurement=yes  SetLabelI=off  LabelI=Iabc  Ipu=off  Pbase=100e6  Vbase=500e3  OutputType=Complex  PhasorSimulation=off  PSBequivalent=0
  Universal Bridge1 : powerlib/Power Electronics/Universal Bridge  Arms=3  SnubberResistance=1e5  SnubberCapacitance=inf  Device=Diodes  Ron=1e-3  Lon=0  ForwardVoltages="[  0  0  ]"  ForwardVoltage=0  GTOparameters=[ 10e-6 , 20e-6 ]  IGBTparameters=[ 1e-6 , 2e-6 ]  Measurements=None  Measurements_2=None  converterType=Rectifier
  Voltage Measurement : powerlib/Measurements/Voltage Measurement  PhasorSimulation=off  OutputType=Complex  PSBequivalent=0
  Series RLC Branch1 : PMIOPort  Side=Left
  Series RLC Branch2 : PMIOPort  Port=2  Side=Left
  Series RLC Branch3 : PMIOPort  Port=3  Side=Left
  wires:
  IGBT/Diode9/1 -> Scopedata131/1
  Three-Phase V-I Measurement2/2 -> Scopedata135/1
  Pulse Generator10/1 -> IGBT/Diode5/1
  Pulse Generator6/1 -> IGBT/Diode11/1
  Pulse Generator7/1 -> IGBT/Diode8/1
  Pulse Generator9/1 -> IGBT/Diode10/1
  Three-Phase V-I Measurement2/1 -> Scopedata135/2
  Pulse Generator8/1 -> IGBT/Diode9/1
  Pulse Generator11/1 -> IGBT/Diode12/1
  IGBT/Diode12/1 -> Scopedata132/1
  IGBT/Diode8/1 -> Scopedata130/1
  IGBT/Diode11/1 -> Scopedata129/1
  IGBT/Diode5/1 -> Scopedata133/1
  IGBT/Diode10/1 -> Scopedata134/1
  Voltage Measurement/1 -> Scope/1
  Current Measurement/1 -> Scope/2
  connections:
  IGBT/Diode9/RConn1 -- IGBT/Diode10/LConn1 -- Three-Phase V-I Measurement2/LConn3
  IGBT/Diode5/RConn1 -- IGBT/Diode10/RConn1 -- IGBT/Diode12/RConn1 -- Current Measurement/RConn1 -- Voltage Measurement/LConn2 -- Universal Bridge1/RConn2
  IGBT/Diode11/RConn1 -- Three-Phase V-I Measurement2/LConn1 -- IGBT/Diode12/LConn1
  Three-Phase V-I Measurement2/RConn2 -- Three-Phase Parallel RLC Load1/LConn2
  IGBT/Diode8/RConn1 -- IGBT/Diode5/LConn1 -- Three-Phase V-I Measurement2/LConn2
  Three-Phase V-I Measurement2/RConn3 -- Three-Phase Parallel RLC Load1/LConn3
  Three-Phase V-I Measurement2/RConn1 -- Three-Phase Parallel RLC Load1/LConn1
  Voltage Measurement/LConn1 -- Series RLC Branch4/RConn1 -- Current Measurement/LConn1 -- IGBT/Diode11/LConn1 -- IGBT/Diode8/LConn1 -- IGBT/Diode9/LConn1
  Series RLC Branch4/LConn1 -- Universal Bridge1/RConn1
  Universal Bridge1/LConn2 -- Series RLC Branch2/RConn1
  Universal Bridge1/LConn1 -- Series RLC Branch1/RConn1
  Universal Bridge1/LConn3 -- Series RLC Branch3/RConn1

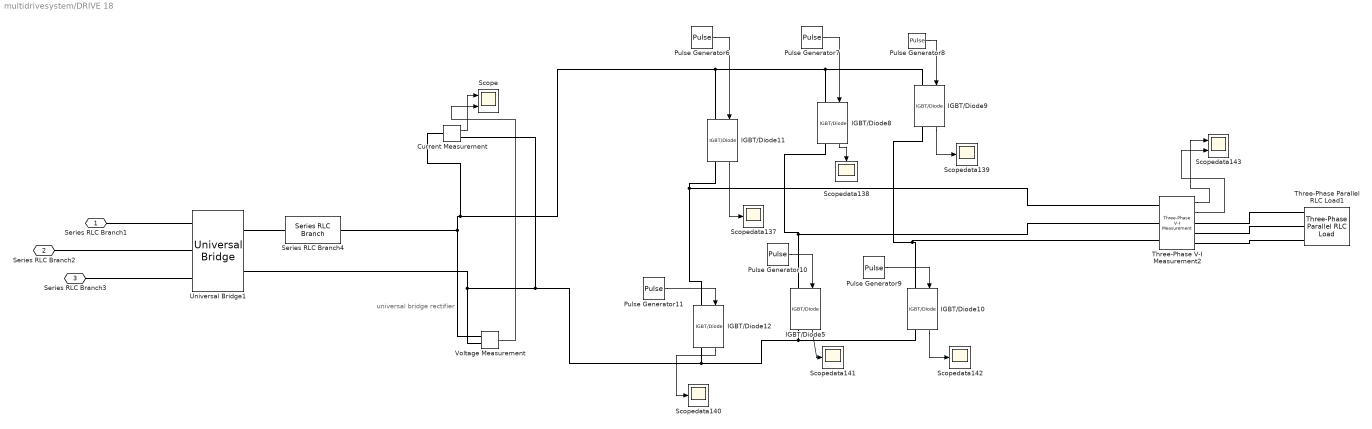
== system multidrivesystem/DRIVE 18 ==
  note: universal bridge rectifier
  Current Measurement : powerlib/Measurements/Current Measurement  PhasorSimulation=off  OutputType=Complex  PSBequivalent=0
  IGBT/Diode{5,8..12} (6 alike) : powerlib/Power Electronics/IGBT//Diode  Ron=1e-3  Rs=1e5  Cs=inf  Measurements=on
  Pulse Generator{6..11} (6 alike) : DiscretePulseGenerator  PulseType=Time based  Period=10  PulseWidth=5
  Scope : Scope  NumInputPorts=2
  Scopedata{137..142} (6 alike) : Scope
  Scopedata143 : Scope  NumInputPorts=2
  Series RLC Branch4 : powerlib/Elements/Series RLC Branch  LConnTagsString=__new0  RConnTagsString=__new0  BranchType=L  Resistance=1  Inductance=3e-3  SetiL0=off  InitialCurrent=0  Capacitance=1e-6  Setx0=off  InitialVoltage=0  Measurements=None
  Three-Phase Parallel RLC Load1 : powerlib/Elements/Three-Phase Parallel RLC Load  LConnTagsString=A|B|C  Configuration=Y (grounded)  NominalVoltage=1000  Vabc=[1e3 1e3 1e3]  Vabcp=[1e3 1e3 1e3]  NominalFrequency=60  UnbalancedPower=off  ActivePower=8e3  InductivePower=0  CapacitivePower=0  Pabc=[10e3 9e3 11e3]  QLabc=[100 90 110]  QCabc=[100 90 110]  Pabcp=[10e3 9e3 11e3]  QLabcp=[100 90 110]  QCabcp=[100 90 110]  Measurements=None  LoadType=constant Z
  Three-Phase V-I Measurement2 : powerlib/Measurements/Three-Phase V-I Measurement  VoltageMeasurement=phase-to-ground  SetLabelV=off  LabelV=Vabc  Vpu=off  VpuLL=off  CurrentMeasurement=yes  SetLabelI=off  LabelI=Iabc  Ipu=off  Pbase=100e6  Vbase=500e3  OutputType=Complex  PhasorSimulation=off  PSBequivalent=0
  Universal Bridge1 : powerlib/Power Electronics/Universal Bridge  Arms=3  SnubberResistance=1e5  SnubberCapacitance=inf  Device=Diodes  Ron=1e-3  Lon=0  ForwardVoltages="[  0  0  ]"  ForwardVoltage=0  GTOparameters=[ 10e-6 , 20e-6 ]  IGBTparameters=[ 1e-6 , 2e-6 ]  Measurements=None  Measurements_2=None  converterType=Rectifier
  Voltage Measurement : powerlib/Measurements/Voltage Measurement  PhasorSimulation=off  OutputType=Complex  PSBequivalent=0
  Series RLC Branch1 : PMIOPort  Side=Left
  Series RLC Branch2 : PMIOPort  Port=2  Side=Left
  Series RLC Branch3 : PMIOPort  Port=3  Side=Left
  wires:
  IGBT/Diode10/1 -> Scopedata142/1
  IGBT/Diode5/1 -> Scopedata141/1
  IGBT/Diode11/1 -> Scopedata137/1
  IGBT/Diode8/1 -> Scopedata138/1
  IGBT/Diode12/1 -> Scopedata140/1
  Pulse Generator11/1 -> IGBT/Diode12/1
  Pulse Generator8/1 -> IGBT/Diode9/1
  Three-Phase V-I Measurement2/1 -> Scopedata143/1
  Pulse Generator9/1 -> IGBT/Diode10/1
  Pulse Generator7/1 -> IGBT/Diode8/1
  Pulse Generator6/1 -> IGBT/Diode11/1
  Pulse Generator10/1 -> IGBT/Diode5/1
  Three-Phase V-I Measurement2/2 -> Scopedata143/2
  IGBT/Diode9/1 -> Scopedata139/1
  Current Measurement/1 -> Scope/1
  Voltage Measurement/1 -> Scope/2
  connections:
  Three-Phase V-I Measurement2/RConn1 -- Three-Phase Parallel RLC Load1/LConn1
  Three-Phase V-I Measurement2/RConn3 -- Three-Phase Parallel RLC Load1/LConn3
  Three-Phase V-I Measurement2/LConn2 -- IGBT/Diode5/LConn1 -- IGBT/Diode8/RConn1
  Three-Phase V-I Measurement2/RConn2 -- Three-Phase Parallel RLC Load1/LConn2
  IGBT/Diode12/LConn1 -- Three-Phase V-I Measurement2/LConn1 -- IGBT/Diode11/RConn1
  IGBT/Diode12/RConn1 -- IGBT/Diode10/RConn1 -- IGBT/Diode5/RConn1 -- Current Measurement/RConn1 -- Voltage Measurement/LConn2 -- Universal Bridge1/RConn2
  Three-Phase V-I Measurement2/LConn3 -- IGBT/Diode10/LConn1 -- IGBT/Diode9/RConn1
  Current Measurement/LConn1 -- Series RLC Branch4/RConn1 -- Voltage Measurement/LConn1 -- IGBT/Diode9/LConn1 -- IGBT/Diode8/LConn1 -- IGBT/Diode11/LConn1
  Series RLC Branch4/LConn1 -- Universal Bridge1/RConn1
  Universal Bridge1/LConn1 -- Series RLC Branch1/RConn1
  Universal Bridge1/LConn2 -- Series RLC Branch2/RConn1
  Universal Bridge1/LConn3 -- Series RLC Branch3/RConn1

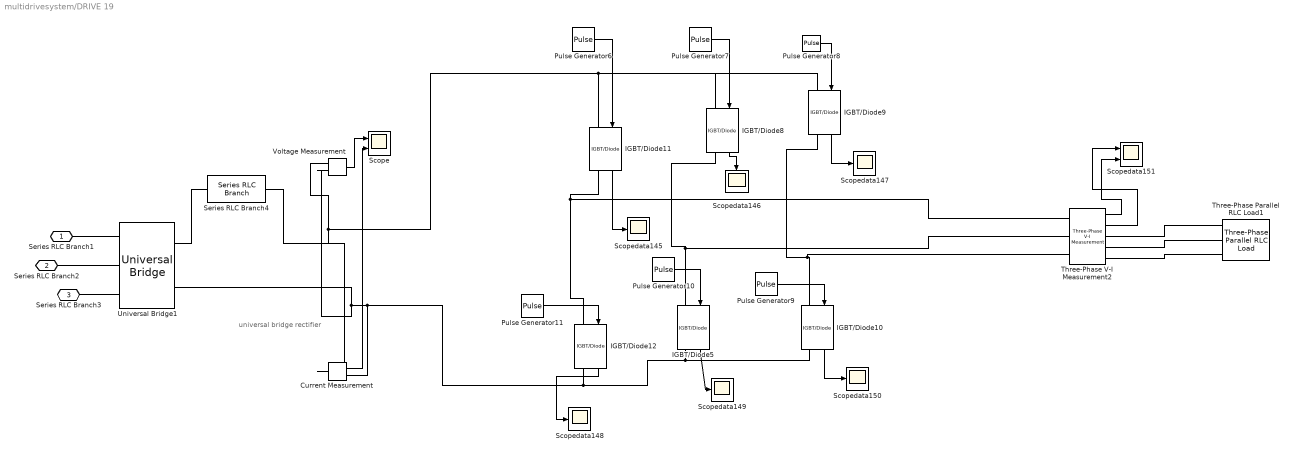
== system multidrivesystem/DRIVE 19 ==
  note: universal bridge rectifier
  Current Measurement : powerlib/Measurements/Current Measurement  PhasorSimulation=off  OutputType=Complex  PSBequivalent=0
  IGBT/Diode{5,8..12} (6 alike) : powerlib/Power Electronics/IGBT//Diode  Ron=1e-3  Rs=1e5  Cs=inf  Measurements=on
  Pulse Generator{6..11} (6 alike) : DiscretePulseGenerator  PulseType=Time based  Period=10  PulseWidth=5
  Scope : Scope  NumInputPorts=2
  Scopedata{145..150} (6 alike) : Scope
  Scopedata151 : Scope  NumInputPorts=2
  Series RLC Branch4 : powerlib/Elements/Series RLC Branch  LConnTagsString=__new0  RConnTagsString=__new0  BranchType=L  Resistance=1  Inductance=3e-3  SetiL0=off  InitialCurrent=0  Capacitance=1e-6  Setx0=off  InitialVoltage=0  Measurements=None
  Three-Phase Parallel RLC Load1 : powerlib/Elements/Three-Phase Parallel RLC Load  LConnTagsString=A|B|C  Configuration=Y (grounded)  NominalVoltage=1000  Vabc=[1e3 1e3 1e3]  Vabcp=[1e3 1e3 1e3]  NominalFrequency=60  UnbalancedPower=off  ActivePower=2e3  InductivePower=0  CapacitivePower=0  Pabc=[10e3 9e3 11e3]  QLabc=[100 90 110]  QCabc=[100 90 110]  Pabcp=[10e3 9e3 11e3]  QLabcp=[100 90 110]  QCabcp=[100 90 110]  Measurements=None  LoadType=constant Z
  Three-Phase V-I Measurement2 : powerlib/Measurements/Three-Phase V-I Measurement  VoltageMeasurement=phase-to-ground  SetLabelV=off  LabelV=Vabc  Vpu=off  VpuLL=off  CurrentMeasurement=yes  SetLabelI=off  LabelI=Iabc  Ipu=off  Pbase=100e6  Vbase=500e3  OutputType=Complex  PhasorSimulation=off  PSBequivalent=0
  Universal Bridge1 : powerlib/Power Electronics/Universal Bridge  Arms=3  SnubberResistance=1e5  SnubberCapacitance=inf  Device=Diodes  Ron=1e-3  Lon=0  ForwardVoltages="[  0  0  ]"  ForwardVoltage=0  GTOparameters=[ 10e-6 , 20e-6 ]  IGBTparameters=[ 1e-6 , 2e-6 ]  Measurements=None  Measurements_2=None  converterType=Rectifier
  Voltage Measurement : powerlib/Measurements/Voltage Measurement  PhasorSimulation=off  OutputType=Complex  PSBequivalent=0
  Series RLC Branch1 : PMIOPort  Side=Left
  Series RLC Branch2 : PMIOPort  Port=2  Side=Left
  Series RLC Branch3 : PMIOPort  Port=3  Side=Left
  wires:
  IGBT/Diode9/1 -> Scopedata147/1
  Three-Phase V-I Measurement2/2 -> Scopedata151/1
  Pulse Generator10/1 -> IGBT/Diode5/1
  Pulse Generator6/1 -> IGBT/Diode11/1
  Pulse Generator7/1 -> IGBT/Diode8/1
  Pulse Generator9/1 -> IGBT/Diode10/1
  Three-Phase V-I Measurement2/1 -> Scopedata151/2
  Pulse Generator8/1 -> IGBT/Diode9/1
  Pulse Generator11/1 -> IGBT/Diode12/1
  IGBT/Diode12/1 -> Scopedata148/1
  IGBT/Diode8/1 -> Scopedata146/1
  IGBT/Diode11/1 -> Scopedata145/1
  IGBT/Diode5/1 -> Scopedata149/1
  IGBT/Diode10/1 -> Scopedata150/1
  Voltage Measurement/1 -> Scope/1
  Current Measurement/1 -> Scope/2
  connections:
  Voltage Measurement/LConn1 -- Series RLC Branch4/RConn1 -- Current Measurement/LConn1 -- IGBT/Diode11/LConn1 -- IGBT/Diode8/LConn1 -- IGBT/Diode9/LConn1
  IGBT/Diode9/RConn1 -- IGBT/Diode10/LConn1 -- Three-Phase V-I Measurement2/LConn3
  IGBT/Diode5/RConn1 -- IGBT/Diode10/RConn1 -- IGBT/Diode12/RConn1 -- Current Measurement/RConn1 -- Voltage Measurement/LConn2 -- Universal Bridge1/RConn2
  IGBT/Diode11/RConn1 -- Three-Phase V-I Measurement2/LConn1 -- IGBT/Diode12/LConn1
  Three-Phase V-I Measurement2/RConn2 -- Three-Phase Parallel RLC Load1/LConn2
  IGBT/Diode8/RConn1 -- IGBT/Diode5/LConn1 -- Three-Phase V-I Measurement2/LConn2
  Three-Phase V-I Measurement2/RConn3 -- Three-Phase Parallel RLC Load1/LConn3
  Three-Phase V-I Measurement2/RConn1 -- Three-Phase Parallel RLC Load1/LConn1
  Series RLC Branch1/RConn1 -- Universal Bridge1/LConn1
  Series RLC Branch2/RConn1 -- Universal Bridge1/LConn2
  Series RLC Branch3/RConn1 -- Universal Bridge1/LConn3
  Series RLC Branch4/LConn1 -- Universal Bridge1/RConn1
